simulink model "CONTROL"  (R2023b)
settings: Solver=VariableStepAuto  StartTime=0.0  StopTime=10.0  RelTol=1e-3
settings Model: Creator=lucaerviati  LastModifiedBy=carol
settings DataIOCC: SaveOutput=off  SaveTime=off
settings OptimizationCC: ReuseModelBlockBuffer=off
settings GRTTargetCC: CombineOutputUpdateFcns=off  MatFileLogging=off

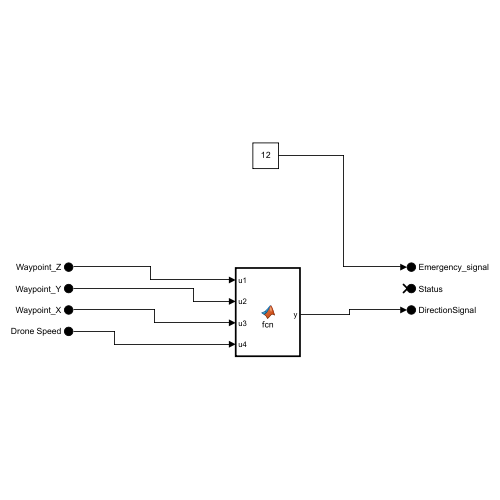
[thumbnail: Simulink's stored preview of the top-level diagram]
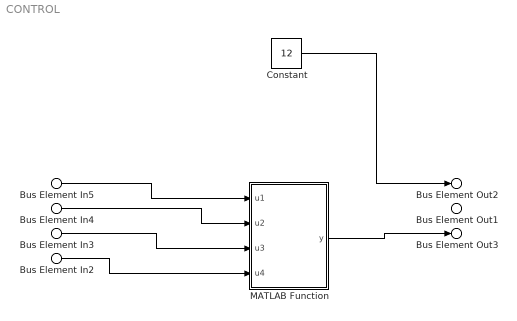
== system CONTROL ==
  Bus Element In5 : Inport  PortName=Waypoint_Z
  Bus Element In4 : Inport  Port=2  PortName=Waypoint_Y
  Bus Element In3 : Inport  Port=3  PortName=Waypoint_X
  Bus Element In2 : Inport  Port=4  PortName=Drone Speed
  Constant : Constant  Value=12
  MATLAB Function : MATLAB Function  TreatAsAtomicUnit=on
  Bus Element Out2 : Outport  PortName=Emergency_signal
  Bus Element Out1 : Outport  Port=2  PortName=Status
  Bus Element Out3 : Outport  Port=3  PortName=DirectionSignal
  wires:
  Constant/1 -> Bus Element Out2/1
  MATLAB Function/1(y) -> Bus Element Out3/1
  Bus Element In5/1 -> MATLAB Function/1(u1)
  Bus Element In4/1 -> MATLAB Function/2(u2)
  Bus Element In3/1 -> MATLAB Function/3(u3)
  Bus Element In2/1 -> MATLAB Function/4(u4)

== matlab function CONTROL/MATLAB Function ==
  data: u1 input; y output; u2 input; u3 input; u4 input
function y = fcn(u1,u2,u3,u4)

u = [10,10,10,10];
y = u;
end
